simulink model "Elevator"  (R2024b)
settings: Solver=VariableStepAuto  StartTime=0.0  StopTime=inf  RelTol=1e-3
settings Model: Creator=madzz  LastModifiedBy=madzz

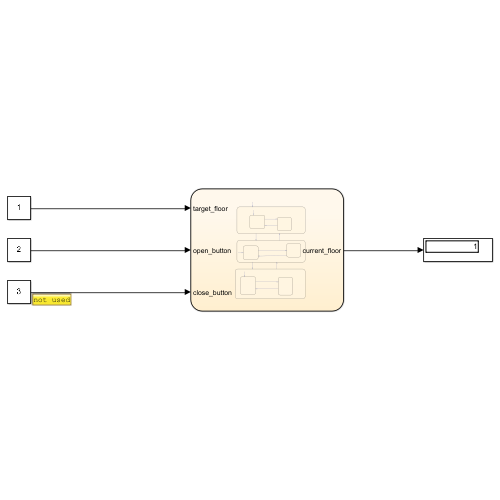
[thumbnail: Simulink's stored preview of the top-level diagram]
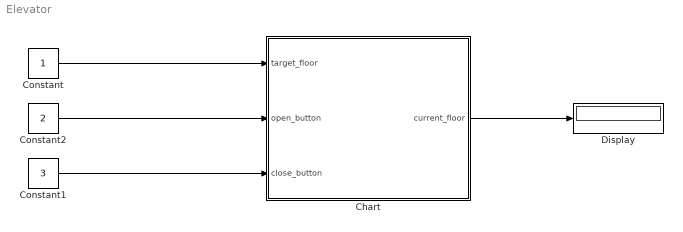
== system Elevator ==
  Chart : Stateflow chart  TreatAsAtomicUnit=on
  Constant : Constant
  Constant1 : Constant  Value=3
  Constant2 : Constant  Value=2
  Display : Display
  wires:
  Constant/1 -> Chart/1(target_floor)
  Constant1/1 -> Chart/3(close_button)
  Constant2/1 -> Chart/2(open_button)
  Chart/1(current_floor) -> Display/1

== stateflow chart Elevator/Chart ==
  state floor_1
    current_floor = 1;  % For Floor 1
    state door_closed
    state door_open
    (default) -> floor_1.door_closed
    floor_1.door_closed -> floor_1.door_open : [open_button == 1
        | ]
    floor_1.door_open -> floor_1.door_closed : [close_button == 1
        | ]
  state floor_2
    current_floor = 2;  % For Floor 2
    state door_open
    state door_closed
    floor_2.door_closed -> floor_2.door_open : [open_button == 1
        | ]
    (default) -> floor_2.door_closed
    floor_2.door_open -> floor_2.door_closed : [close_button == 1
        | ]
  state floor_3
    current_floor = 3;  % For Floor 3
    state door_closed
    state door_open
    (default) -> floor_3.door_closed
    floor_3.door_closed -> floor_3.door_open : [open_button == 1
        | ]
    floor_3.door_open -> floor_3.door_closed : [close_button == 1
        | ]
  (default) -> floor_1
  floor_1 -> floor_2 : [target_floor == 2
      | ]
  floor_2 -> floor_1 [order 1] : [target_floor == 1]
  floor_2 -> floor_3 [order 2] : [target_floor == 3]
  floor_3 -> floor_2 : [target_floor == 2]
  data: target_floor input; current_floor output; open_button input; close_button input
